simulink model "Section2_v"  (R2023b)
settings: Solver=VariableStepAuto  StartTime=0.0  StopTime=10.0  RelTol=1e-3
settings Model: Creator=paria  LastModifiedBy=paria

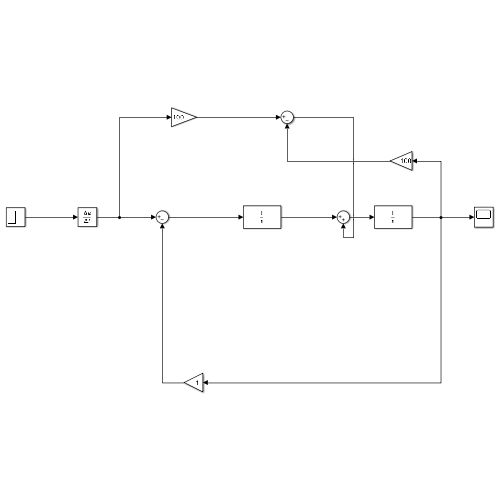
[thumbnail: Simulink's stored preview of the top-level diagram]
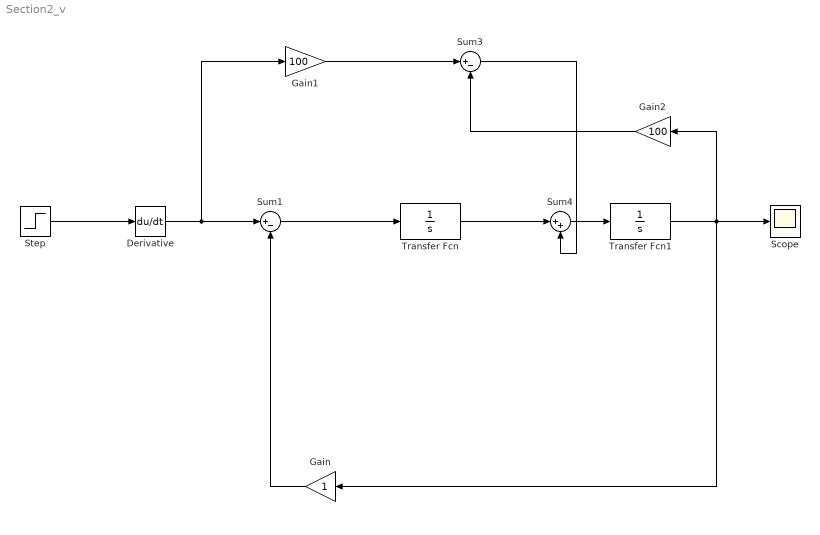
== system Section2_v ==
  Derivative : Derivative
  Gain : Gain
  Gain1 : Gain  Gain=100
  Gain2 : Gain  Gain=100
  Scope : Scope
  Step : Step  Time=0.001  SampleTime=0
  Sum1 : Sum  Inputs=|+-
  Sum3 : Sum  Inputs=|+-
  Sum4 : Sum  Inputs=|++
  Transfer Fcn : TransferFcn  Denominator=[1 0]
  Transfer Fcn1 : TransferFcn  Denominator=[1 0]
  wires:
  Derivative/1 -> Gain1/1, Sum1/1
  Sum3/1 -> Sum4/2
  Step/1 -> Derivative/1
  Transfer Fcn1/1 -> Gain2/1, Scope/1, Gain/1
  Transfer Fcn/1 -> Sum4/1
  Gain2/1 -> Sum3/2
  Gain1/1 -> Sum3/1
  Sum1/1 -> Transfer Fcn/1
  Sum4/1 -> Transfer Fcn1/1
  Gain/1 -> Sum1/2
